simulink model "CarQuarter"  (R2018b)
settings: Solver=VariableStepAuto  StartTime=0.0  StopTime=1000  RelTol=1e-3
settings Model: Creator=Reece Bell  LastModifiedBy=Reece Bell

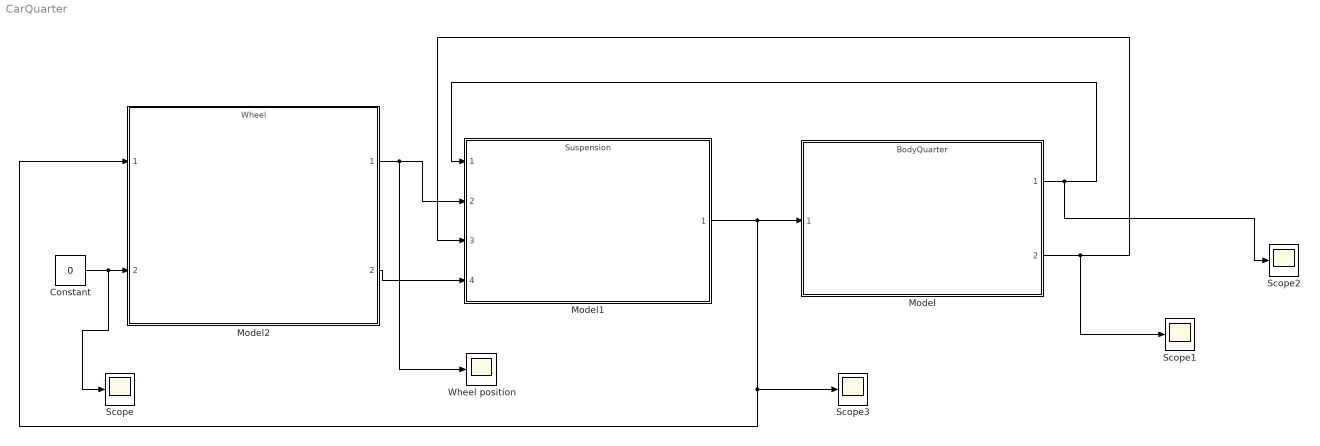
== system CarQuarter ==
  Constant : Constant  Value=0
  Model : ModelReference  ModelNameDialog=BodyQuarter.slx  SimulationMode=Normal  ModelReferenceVersion=1.11
  Model1 : ModelReference  ModelNameDialog=Suspension.slx  SimulationMode=Normal  ModelReferenceVersion=1.4
  Model2 : ModelReference  ModelNameDialog=Wheel.slx  SimulationMode=Normal  ModelReferenceVersion=1.11
  Scope{,1..3} (4 alike) : Scope
  Wheel position : Scope
  wires:
  Model1/1 -> Model2/1, Scope3/1, Model/1
  Constant/1 -> Scope/1, Model2/2
  Model2/2 -> Model1/4
  Model2/1 -> Wheel position/1, Model1/2
  Model/1 -> Scope2/1, Model1/1
  Model/2 -> Scope1/1, Model1/3
